simulink model "zawieszenie"  (R2018b)
settings: Solver=VariableStepAuto  StartTime=0.0  StopTime=10.0  RelTol=1e-3
values from neighbouring files (symbols this model uses):
  cc = 15000    [zawieszenie_dane.m]
  cw = 200000    [zawieszenie_dane.m]
  dc = 200    [zawieszenie_dane.m]
  dw = 10    [zawieszenie_dane.m]
  mc = 250    [zawieszenie_dane.m]
  mw = 30    [zawieszenie_dane.m]
settings Model: Creator=Kasia  LastModifiedBy=Kasia

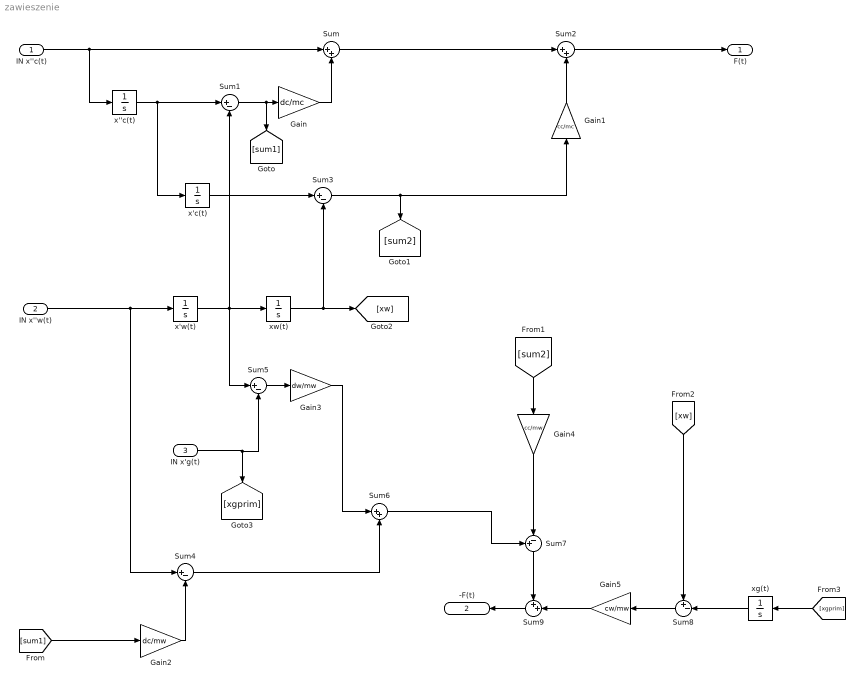
== system zawieszenie ==
  "IN x''c(t) " : Inport
  IN x''w(t) : Inport  Port=2
  IN x'g(t) : Inport  Port=3
  Gain : Gain  Gain=dc/mc
  Gain1 : Gain  Gain=cc/mc
  Gain2 : Gain  Gain=dc/mw
  Gain3 : Gain  Gain=dw/mw
  Gain4 : Gain  Gain=cc/mw
  Gain5 : Gain  Gain=cw/mw
  Sum : Sum  Inputs=|++
      settings: AttributesFormatString=x''c(t)+dc/mc(x'c(t)-x'w(t))
  Sum{1,3..5} (4 alike) : Sum  Inputs=|+-
      Sum1 settings: AttributesFormatString=x'c(t)-x'w(t)
      Sum3 settings: AttributesFormatString=xc(t)-xw(t)
      Sum4 settings: AttributesFormatString=x''w(t)-dc/mw(x'c(t)-x'w(t))
      Sum5 settings: AttributesFormatString=x'w(t)-x'g(t)
  Sum2 : Sum  Inputs=|++
  Sum6 : Sum  Inputs=|++
      settings: AttributesFormatString=x''w(t)-dc/mw(x'c(t)-x'w(t))+dw/mw(x'w(t)-x'g(t))
  Sum7 : Sum  Inputs=+-|
  Sum8 : Sum  Inputs=+-|
      settings: AttributesFormatString=xw(t)-xg(t)
  Sum9 : Sum  Inputs=++|
  x''c(t) : Integrator
  "x'c(t) " : Integrator
  x'w(t) : Integrator
  xg(t) : Integrator
  xw(t) : Integrator
  F(t) : Outport
  -F(t) : Outport  Port=2
  wires:
  "IN x''c(t) "/1 -> Sum/1, x''c(t)/1
  Gain/1 -> Sum/2
  Sum1/1 -> Gain/1, [sum1]
  x''c(t)/1 -> Sum1/1, "x'c(t) "/1
  Sum/1 -> Sum2/1
  Gain1/1 -> Sum2/2
  "x'c(t) "/1 -> Sum3/1
  Sum3/1 -> [sum2], Gain1/1
  Sum2/1 -> F(t)/1
  IN x''w(t)/1 -> Sum4/1, x'w(t)/1
  xw(t)/1 -> [xw], Sum3/2
  x'w(t)/1 -> Sum1/2, xw(t)/1, Sum5/1
  Gain2/1 -> Sum4/2
  [sum1] -> Gain2/1
  IN x'g(t)/1 -> Sum5/2, [xgprim]
  Sum5/1 -> Gain3/1
  Sum4/1 -> Sum6/2
  Gain3/1 -> Sum6/1
  [sum2] -> Gain4/1
  Sum6/1 -> Sum7/1
  Gain4/1 -> Sum7/2
  Sum8/1 -> Gain5/1
  [xw] -> Sum8/1
  [xgprim] -> xg(t)/1
  xg(t)/1 -> Sum8/2
  Gain5/1 -> Sum9/2
  Sum7/1 -> Sum9/1
  Sum9/1 -> -F(t)/1
